simulink library "CTRL_TRGT_SAUPPB"  (R2023b)
settings: Solver=VariableStepAuto  StartTime=0.0  StopTime=10.0  RelTol=1e-3
undefined symbols (not defined in the file or in its folder): c_GravConst_mps2, CTRL_TRGT_SAUPPB_p_Fct1_na
settings Model: Creator=blatak  LastModifiedBy=blatak

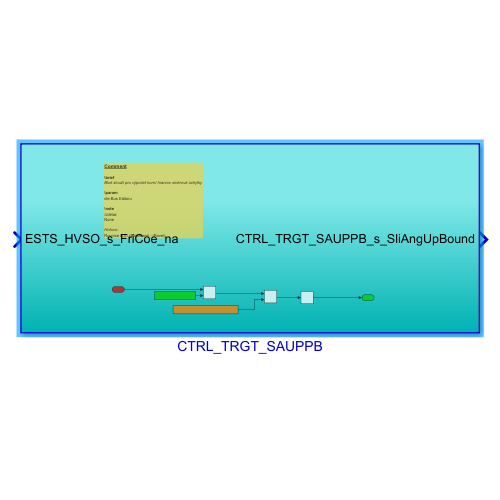
[thumbnail: Simulink's stored preview of the top-level diagram]
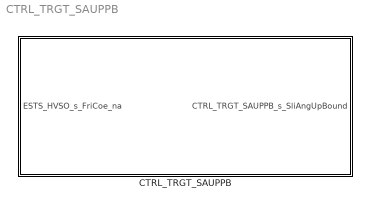
== system CTRL_TRGT_SAUPPB ==
  CTRL_TRGT_SAUPPB : Subsystem

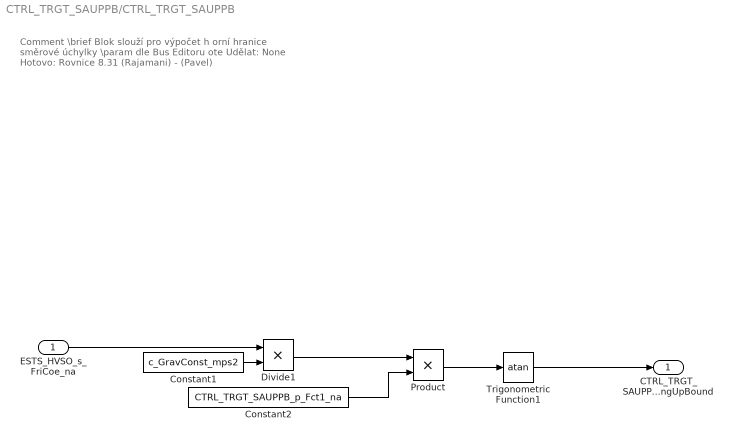
== system CTRL_TRGT_SAUPPB/CTRL_TRGT_SAUPPB ==
  note: Comment
      |
      | \brief
      | Blok slouží pro výpočet h orní hranice směrové úchylky
      |
      | \param
      | dle Bus Editoru
      |
      | \note
      | Udělat:
      | None
      |
      | Hotovo:
      | Rovnice 8.31 (Rajamani) - (Pavel)
  ESTS_HVSO_s_FriCoe_na : Inport
  Constant1 : Constant  Value=c_GravConst_mps2
  Constant2 : Constant  Value=CTRL_TRGT_SAUPPB_p_Fct1_na
  Divide1 : Product  Inputs=**
  Product : Product
  Trigonometric Function1 : Trigonometry  Operator=atan
  CTRL_TRGT_SAUPPB_s_SliAngUpBound : Outport
  wires:
  ESTS_HVSO_s_FriCoe_na/1 -> Divide1/1
  Constant1/1 -> Divide1/2
  Divide1/1 -> Product/1
  Product/1 -> Trigonometric Function1/1
  Trigonometric Function1/1 -> CTRL_TRGT_SAUPPB_s_SliAngUpBound/1
  Constant2/1 -> Product/2
